simulink model "operatorhaschanged"  (R2023a)
settings: Solver=FixedStepDiscrete  StartTime=0.0  StopTime=10.0  FixedStep=1  RelTol=1e-3
libraries: simulink x1
settings Model: Creator=Egypt_Laptop  LastModifiedBy=Egypt_Laptop

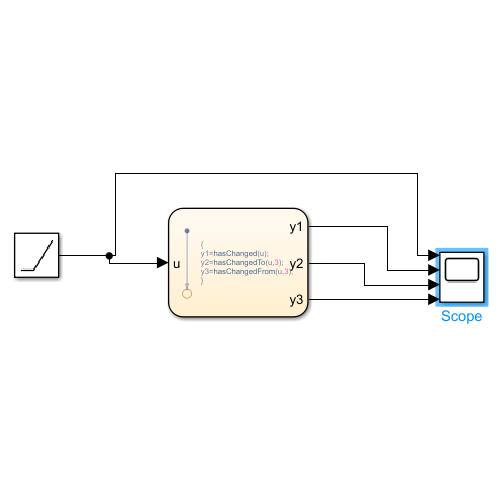
[thumbnail: Simulink's stored preview of the top-level diagram]
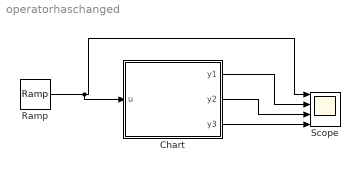
== system operatorhaschanged ==
  Chart : Stateflow chart  TreatAsAtomicUnit=on
  Ramp : simulink/Sources/Ramp  slope=1  start=0  InitialOutput=0
  Scope : Scope  NumInputPorts=4
  wires:
  Chart/1(y1) -> Scope/2
  Chart/2(y2) -> Scope/3
  Chart/3(y3) -> Scope/4
  Ramp/1 -> Chart/1(u), Scope/1

== stateflow chart operatorhaschanged/Chart ==
  (default) -> (junction 5) : {
      | y1=hasChanged(u);
      | y2=hasChangedTo(u,3);
      | y3=hasChangedFrom(u,3);
      | }
  data: y1 output double; y2 output double; y3 output double; u input double
